simulink model "modified_DDPG_ACC"  (R2021b)
settings: Solver=FixedStepAuto  StartTime=0.0  StopTime=Inf  RelTol=1e-3
values from neighbouring files (symbols this model uses):
  amax_ego = 3    [ACC_Integration.m]    (also in AdaptiveCruiseControlExample.m = 2; SAC_agent.m)
  amin_ego = -3    [ACC_Integration.m]    (also in AdaptiveCruiseControlExample.m; SAC_agent.m)
  t_gap = 1.4    [ACC_Integration.m]    (also in SAC_agent.m)
  Ts = 0.1    [ACC_Integration.m]    (also in AdaptiveCruiseControlExample.m; SAC_agent.m)
  v0_ego = 20    [ACC_Integration.m]    (also in AdaptiveCruiseControlExample.m; SAC_agent.m)
  v0_lead = 25    [ACC_Integration.m]    (also in AdaptiveCruiseControlExample.m; SAC_agent.m)
  v_set = 30    [ACC_Integration.m]    (also in AdaptiveCruiseControlExample.m; SAC_agent.m)
  x0_ego = 10    [ACC_Integration.m]    (also in AdaptiveCruiseControlExample.m; SAC_agent.m)
  x0_lead = 50    [ACC_Integration.m]    (also in AdaptiveCruiseControlExample.m; SAC_agent.m)
libraries: simulink x7, mpcadaslib x1, rllib x1
settings Model: Creator=The MathWorks, Inc.  LastModifiedBy=awihb
settings SolverCC: AlgebraicLoopSolver=TrustRegion
settings DebuggingCC: SFMachineParentedDataDiag=warning  ArithmeticOperatorsInVariantConditions=warning
settings SFSimCC: SimUseLocalCustomCode=off
settings RTWCC: RTWUseLocalCustomCode=off
settings CodeAppCC: StateflowObjectComments=on

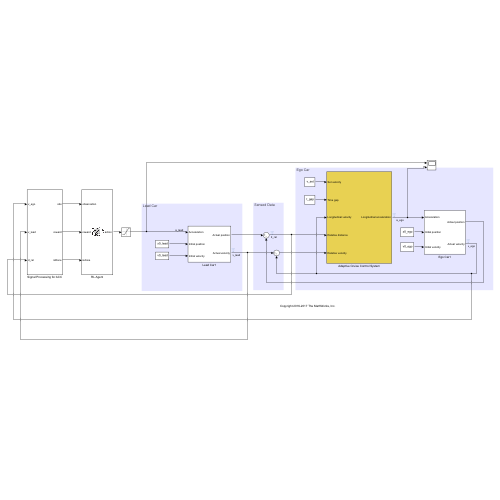
[thumbnail: Simulink's stored preview of the top-level diagram]
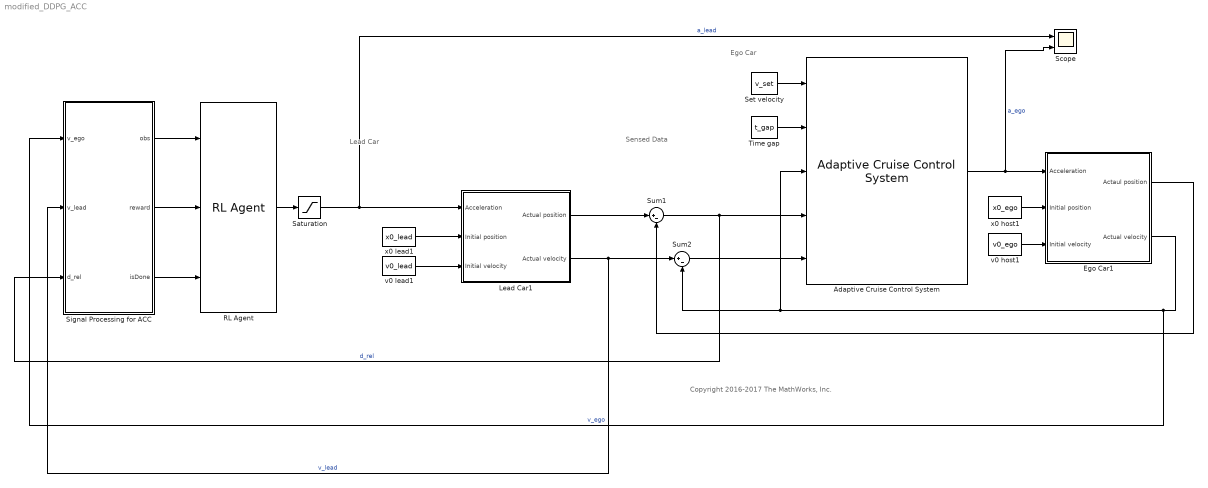
== system modified_DDPG_ACC ==
  note: Sensed Data
  note: Ego Car
  note: Lead Car
  note: Copyright 2016-2017 The MathWorks, Inc.
  Adaptive Cruise Control System : mpcadaslib/Adaptive Cruise Control System  EgoModel=tf(1,[0.5,1,0])  InitialEgoVelocity=20  DefaultSpacing=10  MaxVelocity=50  MinAcceleration=-3  amin_ext=off  MaxAcceleration=3  amax_ext=off  Ts=0.1  PredictionHorizon=30  ControllerBehavior=0.5  suboptimal=off  maxiter=10  datatypeopt=double  optmode=off  trackmode=off
  Ego Car1 : Subsystem
  Lead Car1 : Subsystem
  RL Agent : rllib/RL Agent  Agent=agent  ExternalActionAsInput=off  ProvideCumRwd=off  TreatAsDirectFeedthrough=on
      settings: SourceProductName=Reinforcement Learning
  Saturation : Saturate  UpperLimit=amax_ego  LowerLimit=amin_ego
  Scope : Scope  NumInputPorts=2
  Set velocity : Constant  Value=v_set  SampleTime=Ts
  Signal Processing for ACC : Subsystem
  Sum1 : Sum  Inputs=|+-
  Sum2 : Sum  Inputs=|+-
  Time gap : Constant  Value=t_gap  SampleTime=Ts
  v0 host1 : Constant  Value=v0_ego  SampleTime=Ts
  v0 lead1 : Constant  Value=v0_lead  SampleTime=Ts
  x0 host1 : Constant  Value=x0_ego  SampleTime=Ts
  x0 lead1 : Constant  Value=x0_lead  SampleTime=Ts
  wires:
  Signal Processing for ACC/2(reward) -> RL Agent/2
  RL Agent/1 -> Saturation/1
  Signal Processing for ACC/3(isDone) -> RL Agent/3
  Signal Processing for ACC/1(obs) -> RL Agent/1
  Sum2/1 -> Adaptive Cruise Control System/5
  Time gap/1 -> Adaptive Cruise Control System/2
  Saturation/1 -> Scope/1, Lead Car1/1(Acceleration)  "a_lead"
  Lead Car1/2(Actual velocity) -> Signal Processing for ACC/2(v_lead), Sum2/1  "v_lead"
  Sum1/1 -> Signal Processing for ACC/3(d_rel), Adaptive Cruise Control System/4  "d_rel"
  Lead Car1/1(Actual position) -> Sum1/1
  Set velocity/1 -> Adaptive Cruise Control System/1
  v0 lead1/1 -> Lead Car1/3(Initial velocity)
  Ego Car1/1(Actaul position) -> Sum1/2
  v0 host1/1 -> Ego Car1/3(Initial velocity)
  x0 lead1/1 -> Lead Car1/2(Initial position)
  Ego Car1/2(Actual velocity) -> Signal Processing for ACC/1(v_ego), Adaptive Cruise Control System/3, Sum2/2  "v_ego"
  Adaptive Cruise Control System/1 -> Scope/2, Ego Car1/1(Acceleration)  "a_ego"
  x0 host1/1 -> Ego Car1/2(Initial position)

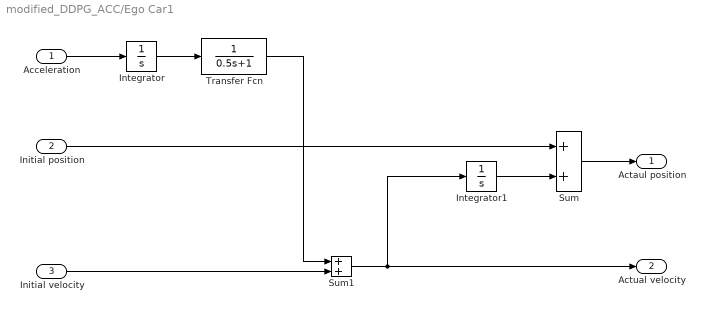
== system modified_DDPG_ACC/Ego Car1 ==
  Acceleration : Inport
  Initial position : Inport  Port=2
  Initial velocity : Inport  Port=3
  Integrator : Integrator
  Integrator1 : Integrator
  Sum : Sum
  Sum1 : Sum
  Transfer Fcn : TransferFcn  Denominator=[0.5 1]
  Actaul position : Outport  VectorParamsAs1DForOutWhenUnconnected=off
  Actual velocity : Outport  Port=2  VectorParamsAs1DForOutWhenUnconnected=off
  wires:
  Sum1/1 -> Integrator1/1, Actual velocity/1
  Initial velocity/1 -> Sum1/2
  Sum/1 -> Actaul position/1
  Transfer Fcn/1 -> Sum1/1
  Integrator/1 -> Transfer Fcn/1
  Acceleration/1 -> Integrator/1
  Initial position/1 -> Sum/1
  Integrator1/1 -> Sum/2

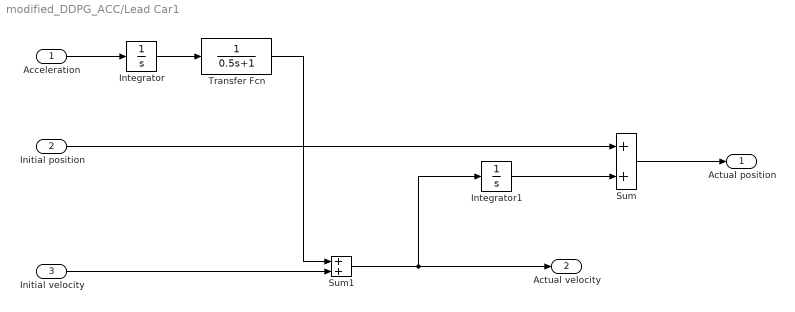
== system modified_DDPG_ACC/Lead Car1 ==
  Acceleration : Inport
  Initial position : Inport  Port=2
  Initial velocity : Inport  Port=3
  Integrator : Integrator
  Integrator1 : Integrator
  Sum : Sum
  Sum1 : Sum
  Transfer Fcn : TransferFcn  Denominator=[0.5 1]
  Actual position : Outport  VectorParamsAs1DForOutWhenUnconnected=off
  Actual velocity : Outport  Port=2  VectorParamsAs1DForOutWhenUnconnected=off
  wires:
  Transfer Fcn/1 -> Sum1/1
  Initial velocity/1 -> Sum1/2
  Sum/1 -> Actual position/1
  Integrator/1 -> Transfer Fcn/1
  Sum1/1 -> Integrator1/1, Actual velocity/1
  Acceleration/1 -> Integrator/1
  Initial position/1 -> Sum/1
  Integrator1/1 -> Sum/2

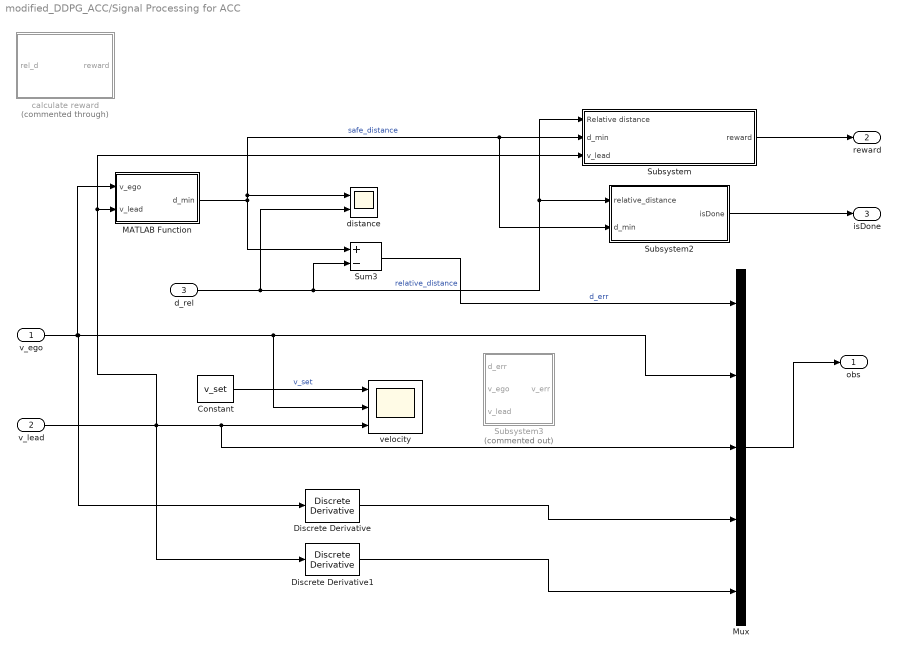
== system modified_DDPG_ACC/Signal Processing for ACC ==
  v_ego : Inport
  v_lead : Inport  Port=2
  d_rel : Inport  Port=3
  Constant : Constant  Value=v_set
  Discrete Derivative : simulink/Discrete/Discrete Derivative  gainval=1.0  ICPrevScaledInput=0.0  OutMin=[]  OutMax=[]  OutDataType=fixdt(1, 16)  OutScaling=2^-10  DoSatur=off
  Discrete Derivative1 : simulink/Discrete/Discrete Derivative  gainval=1.0  ICPrevScaledInput=0.0  OutMin=[]  OutMax=[]  OutDataType=fixdt(1, 16)  OutScaling=2^-10  DoSatur=off
  MATLAB Function : MATLAB Function  TreatAsAtomicUnit=on
  Mux : Mux  Inputs=5
  Subsystem : Subsystem
  Subsystem2 : Subsystem
  Subsystem3 : Subsystem  Commented=on
  Sum3 : Sum  Inputs=+-
  calculate reward : Subsystem  Commented=through
  distance : Scope  NumInputPorts=2
  velocity : Scope  NumInputPorts=3
  obs : Outport  VectorParamsAs1DForOutWhenUnconnected=off
  reward : Outport  Port=2  VectorParamsAs1DForOutWhenUnconnected=off
  isDone : Outport  Port=3  VectorParamsAs1DForOutWhenUnconnected=off
  wires:
  Constant/1 -> velocity/1  "v_set"
  v_lead/1 -> Subsystem/3(v_lead), MATLAB Function/2(v_lead), Mux/3, velocity/3, Discrete Derivative1/1
  Mux/1 -> obs/1
  v_ego/1 -> Discrete Derivative/1, velocity/2, Mux/2, MATLAB Function/1(v_ego)
  d_rel/1 -> distance/2, Subsystem2/1(relative_distance), Subsystem/1(Relative distance), Sum3/2  "relative_distance"
  Sum3/1 -> Mux/1  "d_err"
  MATLAB Function/1(d_min) -> distance/1, Subsystem2/2(d_min), Subsystem/2(d_min), Sum3/1  "safe_distance"
  Subsystem2/1(isDone) -> isDone/1
  Subsystem/1(reward) -> reward/1
  Discrete Derivative/1 -> Mux/4
  Discrete Derivative1/1 -> Mux/5

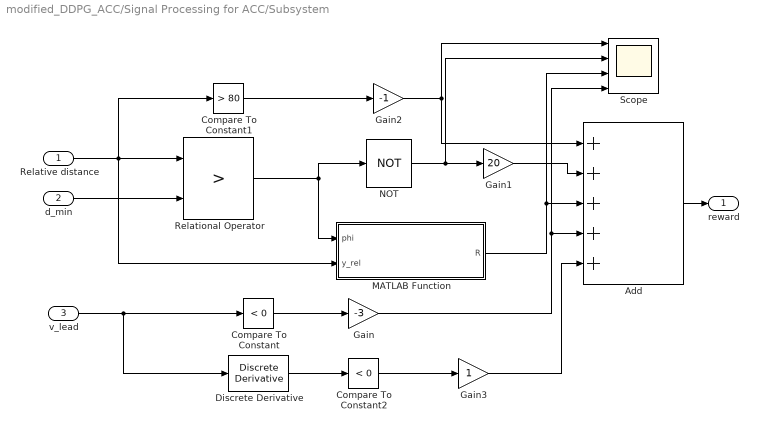
== system modified_DDPG_ACC/Signal Processing for ACC/Subsystem ==
  Relative distance : Inport
  d_min : Inport  Port=2
  v_lead : Inport  Port=3
  Add : Sum  Inputs=+++++
  Compare To Constant : simulink/Logic and Bit Operations/Compare To Constant  relop=<  const=0  OutDataTypeStr=boolean
  Compare To Constant1 : simulink/Logic and Bit Operations/Compare To Constant  relop=>  const=80  OutDataTypeStr=boolean
  Compare To Constant2 : simulink/Logic and Bit Operations/Compare To Constant  relop=<  const=0  OutDataTypeStr=boolean
  Discrete Derivative : simulink/Discrete/Discrete Derivative  gainval=1.0  ICPrevScaledInput=0.0  OutMin=[]  OutMax=[]  OutDataType=fixdt(1, 16)  OutScaling=2^-10  DoSatur=off
  Gain : Gain  Gain=-3
  Gain1 : Gain  Gain=20
  Gain2 : Gain  Gain=-1
  Gain3 : Gain
  MATLAB Function : MATLAB Function  TreatAsAtomicUnit=on
  NOT : Logic  Operator=NOT  IconShape=distinctive  AllPortsSameDT=off  OutDataTypeStr=boolean
  Relational Operator : RelationalOperator  Operator=>  OutDataTypeStr=boolean  RndMeth=Simplest
  Scope : Scope  NumInputPorts=4
  reward : Outport
  wires:
  Relative distance/1 -> Compare To Constant1/1, Relational Operator/1, MATLAB Function/2(y_rel)
  d_min/1 -> Relational Operator/2
  Relational Operator/1 -> NOT/1, MATLAB Function/1(phi)
  Add/1 -> reward/1
  MATLAB Function/1(R) -> Scope/3, Add/3
  v_lead/1 -> Compare To Constant/1, Discrete Derivative/1
  Compare To Constant/1 -> Gain/1
  Gain/1 -> Scope/4, Add/4
  NOT/1 -> Scope/2, Gain1/1
  Gain1/1 -> Add/2
  Compare To Constant1/1 -> Gain2/1
  Gain2/1 -> Scope/1, Add/1
  Discrete Derivative/1 -> Compare To Constant2/1
  Compare To Constant2/1 -> Gain3/1
  Gain3/1 -> Add/5

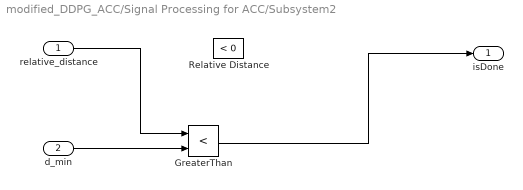
== system modified_DDPG_ACC/Signal Processing for ACC/Subsystem2 ==
  relative_distance : Inport
  d_min : Inport  Port=2
  GreaterThan : RelationalOperator  Operator=<  OutDataTypeStr=boolean  RndMeth=Simplest
  Relative Distance : simulink/Logic and Bit Operations/Compare To Constant  relop=<  const=0  OutDataTypeStr=boolean
  isDone : Outport  VectorParamsAs1DForOutWhenUnconnected=off
  wires:
  relative_distance/1 -> GreaterThan/1
  GreaterThan/1 -> isDone/1
  d_min/1 -> GreaterThan/2

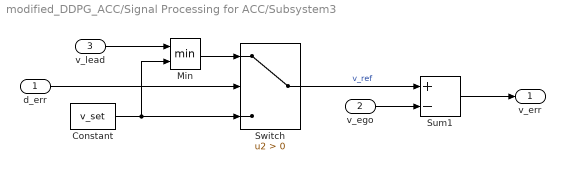
== system modified_DDPG_ACC/Signal Processing for ACC/Subsystem3 ==
  d_err : Inport
  v_ego : Inport  Port=2
  v_lead : Inport  Port=3
  Constant : Constant  Value=v_set
  Min : MinMax  Inputs=2
  Sum1 : Sum  Inputs=+-
  Switch : Switch  Criteria=u2 > Threshold
  v_err : Outport  VectorParamsAs1DForOutWhenUnconnected=off
  wires:
  Sum1/1 -> v_err/1
  v_ego/1 -> Sum1/2
  Switch/1 -> Sum1/1  "v_ref"
  d_err/1 -> Switch/2
  Constant/1 -> Min/2, Switch/3
  Min/1 -> Switch/1
  v_lead/1 -> Min/1

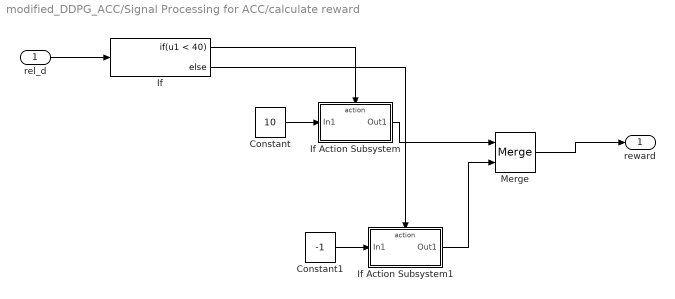
== system modified_DDPG_ACC/Signal Processing for ACC/calculate reward ==
  rel_d : Inport
  Constant : Constant  Value=10
  Constant1 : Constant  Value=-1
  If : If  IfExpression=u1 < 40
  If Action Subsystem : Subsystem  TreatAsAtomicUnit=on
  If Action Subsystem1 : Subsystem  TreatAsAtomicUnit=on
  Merge : Merge
  reward : Outport  VectorParamsAs1DForOutWhenUnconnected=off
  wires:
  rel_d/1 -> If/1
  If/1 -> If Action Subsystem/Action
  Constant/1 -> If Action Subsystem/1(In1)
  Constant1/1 -> If Action Subsystem1/1(In1)
  If/2 -> If Action Subsystem1/Action
  If Action Subsystem/1(Out1) -> Merge/1
  If Action Subsystem1/1(Out1) -> Merge/2
  Merge/1 -> reward/1

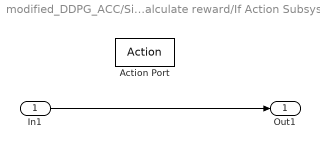
== system modified_DDPG_ACC/Signal Processing for ACC/calculate reward/If Action Subsystem ==
  In1 : Inport
  Action Port : ActionPort
  Out1 : Outport
  wires:
  In1/1 -> Out1/1

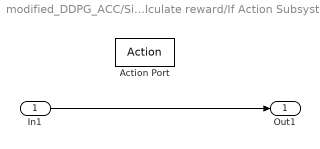
== system modified_DDPG_ACC/Signal Processing for ACC/calculate reward/If Action Subsystem1 ==
  In1 : Inport
  Action Port : ActionPort
  Out1 : Outport
  wires:
  In1/1 -> Out1/1

== matlab function modified_DDPG_ACC/Signal Processing for ACC/MATLAB Function ==
  data: v_ego input; d_min output; v_lead input
function d_min=dmin(v_ego,v_lead)
%To compute the minimum distance
% Response time
tr=0.1;
% Max acceleration of ego car 
a_max_acc=3;
% Max acceleration of lead car to full stop
a_max_brake=-3;
% Min acceleration of lead car to full stop
a_min_brake=-2.5;
temp=v_ego*tr+a_max_acc*tr^2/2 + (v_ego+a_max_acc*tr)^2/(2*a_min_brake) -v_lead^2/(2*a_max_brake);
if temp <0
   d_min=0;
else
   d_min=temp ;
end
end

== matlab function modified_DDPG_ACC/Signal Processing for ACC/Subsystem/MATLAB Function ==
  data: phi input; R output; y_rel input
function R = reward_function(phi,y_rel)
    R = exp(-phi*y_rel) -1;

end
